simulink model "ex_ecg_sigprocessing"  (R2022b)
settings: Solver=VariableStepAuto  StartTime=0.0  StopTime=10  RelTol=1e-3  EnableMultiTasking=on
InitFcn:
  | % load recorded real (sampled from a healthy volunteer)
  | % and synthesized ECG data with Fs = 360 Hz
  | % Setting for generating the synthesized ECG data:
  | % Additive uniformly distributed measurement noise 0.005mV
  | % Standard deviation of heart rate [1 beat per minute]
  | 
  | load('ex_ecgdata360Hz.mat')
  | % ecgdata360Hz_hrmean45 : synthesized ECG signal with mean heart rate 45 bpm
  | % ecgdata360Hz_hrmean60 : synthesized ECG signal with mean heart rate 60 bpm
  | % ecgdata360Hz_hrmean160 : synthesized ECG signal with mean heart rate 160 bpm
  | % ecgdata360Hz_hrmean220 : synthesized ECG signal with mean heart rate 220 bpm
  | % ecgdata360Hz_hrmean82 : recorded real ECG sample from a healthy MathWorks volunteer
  | 
  | fs = 360; % sampling frequency of recorded ECG data Hz
  | 
  | 
  | % Define filter
  | fs_filter = 200; % sampling frequency of the filter
  | fc = [5 26]; % Bandpass Filter Spec [Hz]
  | 
  | fc_bandpass = fc/(1/2*fs_filter); % Normalized freq (Matlab convention)
  | 
  | %N = 256; % Order of filter
  | %b = fir1(N,fc_bandpass);
  | 
  | %
  | WinWidthMS = 80; % ms or 80 ms
  | WinSize = WinWidthMS*fs_filter/1000; % moving average window size 80ms
libraries: dspsrcs4 x5, dspsigops x1, dspfdesign x1, slpidlib x1, sldrtlib x1
CloseFcn:
  | clear fc;
  | clear fc_bandpass;
  | clear fs;
  | clear fs_filter;
  | clear WinWidthMS;
  | clear WinSize;
  | clear ecgdata360Hz_hrmean45;
  | clear ecgdata360Hz_hrmean60;
  | clear ecgdata360Hz_hrmean82;
  | clear ecgdata360Hz_hrmean160;
  | clear ecgdata360Hz_hrmean220;
settings Model: ExtModeTrigDuration=10000  Creator=The MathWorks, Inc.  LastModifiedBy={ AZAN Laptops }
settings SolverCC: AlgebraicLoopSolver=TrustRegion  MaxZcPerStep=1
settings DataIOCC: LimitDataPoints=on  SaveFormat=Array  ReturnWorkspaceOutputs=off
settings OptimizationCC: LifeSpan=1  MaxStackSize=64  SimCompilerOptimization=on  EfficientTunableParamExpr=on
settings DebuggingCC: SolverPrmCheckMsg=warning  ParameterPrecisionLossMsg=none  UnconnectedInputMsg=warning  UnconnectedOutputMsg=warning  UnconnectedLineMsg=warning  AllowSymbolicDim=off  SymbolicDimsDataTypeCodeGenerationDiagnostic=none  SFUnexpectedBacktrackingDiag=warning  SFNoUnconditionalDefaultTransitionDiag=warning  SFExecutionAtInitializationDiag=none  SFMachineParentedDataDiag=warning  ArithmeticOperatorsInVariantConditions=warning
settings HardwareCC: ProdBitPerPointer=32  ProdLargestAtomicInteger=Long  ProdLargestAtomicFloat=Double  ProdIntDivRoundTo=Undefined  ProdWordSize=32  ProdHWDeviceType=ARM Compatible->ARM Cortex
settings ModelReferenceCC: EnableRefExpFcnMdlSchedulingChecks=on  PropagateSignalLabelsOutOfModel=off
settings SFSimCC: SimUseLocalCustomCode=off  MATLABDynamicMemAlloc=off  CustomCodeUndefinedFunction=UseInterfaceOnly
settings RTWCC: Description=Embedded Coder  SystemTargetFile=ert.tlc  TemplateMakefile=ert_default_tmf  RTWUseLocalCustomCode=off  DLArmComputeVersion=19.05
settings CodeAppCC: IgnoreCustomStorageClasses=off  StateflowObjectComments=on
settings ERTTargetCC: MultiwordLength=2048  ERTCustomFileTemplate=example_file_process.tlc  ConvertIfToSwitch=off  SuppressUnreachableDefaultCases=off
settings ConfigComp: CovMetricSettings=dw  CovSaveCumulativeToWorkspaceVar=on  CovSaveSingleToWorkspaceVar=on  CovExternalEMLEnable=off  CovSFcnEnable=off

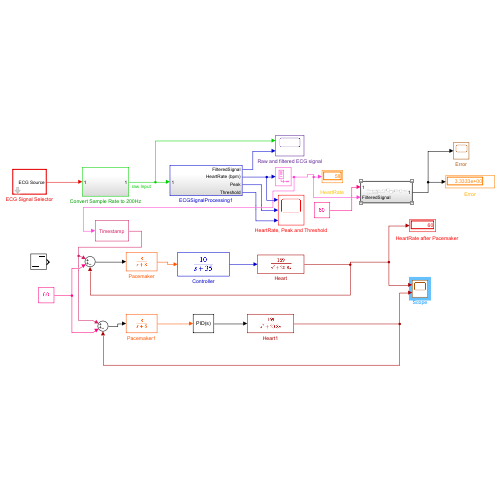
[thumbnail: Simulink's stored preview of the top-level diagram]
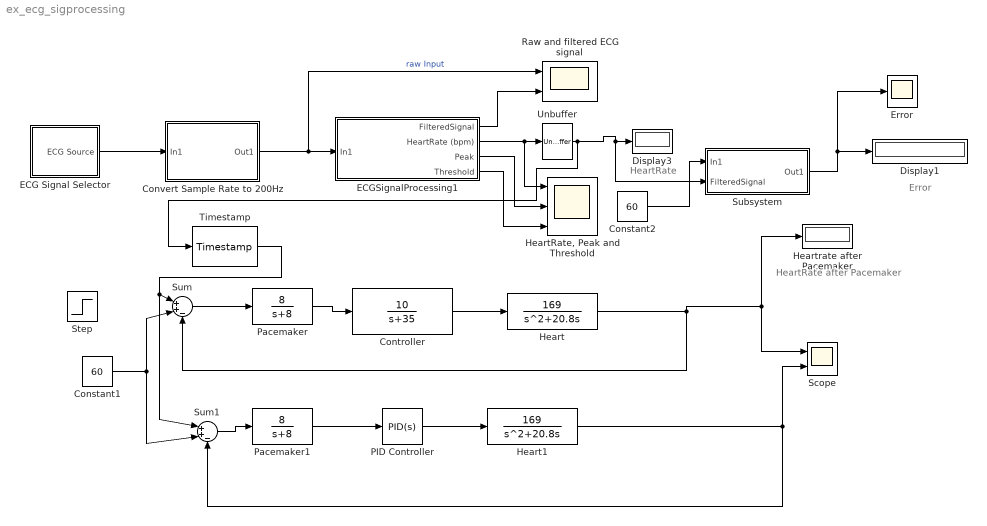
== system ex_ecg_sigprocessing ==
  note: HeartRate
  note: HeartRate after Pacemaker
  note: Error
  Constant1 : Constant  Value=60
  Constant2 : Constant  Value=60
  Controller : TransferFcn  Numerator=[10]  Denominator=[1 35]
  Convert Sample Rate to 200Hz : Subsystem
  Display1 : Display
      settings: Format=short_e
  Display3 : Display
  ECG Signal Selector : Subsystem  TreatAsAtomicUnit=on  mask{K=60 bpm (synthesized)}
      mask prompts: K "Select ECG Signal Mean Heart Rate (Beats Per Minute)"
      mask Help: web(fullfile(docroot,'dsp','examples','real-time-ecg-qrs-detection.html#zmw57dd0e14307'));
      mask TypeOptions K: 45 bpm (synthesized) | 60 bpm (synthesized) | 82 bpm (recorded) | 160 bpm (synthesized) | 220 bpm (synthesized)
  ECGSignalProcessing1 : Subsystem
  Error : Scope
  Heart : TransferFcn  Numerator=[169]  Denominator=[1 20.8 0]
  Heart1 : TransferFcn  Numerator=[169]  Denominator=[1 20.8 0]
  "HeartRate, Peak and Threshold" : Scope  NumInputPorts=3
  "Heartrate after Pacemaker " : Display
  PID Controller : slpidlib/PID Controller  Controller=PID  Form=Parallel  TimeDomain=Continuous-time  UseExternalTs=off  SampleTime=-1  IntegratorMethod=Forward Euler  FilterMethod=Forward Euler  ControllerParametersSource=internal  P=1  I=1  UseKiTs=off  D=0.1  N=100  UseFilter=on  TunerSelectOption=Transfer Function Based (PID Tuner App)  InitialConditionSource=internal  InitialConditionForIntegrator=0  InitialConditionForFilter=0  DifferentiatorICPrevScaledInput=0  ExternalReset=none  TrackingMode=off  Kt=1  LimitOutput=off  SatLimitsSource=internal  UpperSaturationLimit=inf  LowerSaturationLimit=-inf  LinearizeAsGain=on  AntiWindupMode=none  Kb=1  LimitIntegrator=off  UpperIntegratorSaturationLimit=inf  LowerIntegratorSaturationLimit=-inf  POutMin=[]  POutMax=[]  IOutMin=[]  IOutMax=[]  DOutMin=[]  DOutMax=[]  NOutMin=[]  NOutMax=[]  SumOutMin=[]  SumOutMax=[]  SaturationOutMin=[]  SaturationOutMax=[]  PParamMin=[]  PParamMax=[]  IParamMin=[]  IParamMax=[]  DParamMin=[]  DParamMax=[]  NParamMin=[]  NParamMax=[]  KbParamMin=[]  KbParamMax=[]  KtParamMin=[]  KtParamMax=[]  KbOutMin=[]  KbOutMax=[]  KtOutMin=[]  KtOutMax=[]  IntegratorOutMin=[]  IntegratorOutMax=[]  FilterOutMin=[]  FilterOutMax=[]  SumI1OutMin=[]  SumI1OutMax=[]  SumI2OutMin=[]  SumI2OutMax=[]  SumI3OutMin=[]  SumI3OutMax=[]  SumI4OutMin=[]  SumI4OutMax=[]  SumDOutMin=[]  SumDOutMax=[]  DifferentiatorOutMin=[]  DifferentiatorOutMax=[]  FilterDiffOutCoefMin=[]  FilterDiffOutCoefMax=[]  ReciprocalOutMin=[]  ReciprocalOutMax=[]  SumDenOutMin=[]  SumDenOutMax=[]  SumNumOutMin=[]  SumNumOutMax=[]  DivideOutMin=[]  DivideOutMax=[]  UdiffTsProdOutMin=[]  UdiffTsProdOutMax=[]  NTsProdOutMin=[]  NTsProdOutMax=[]  UintegralTsProdOutMin=[]  UintegralTsProdOutMax=[]  UngainTsProdOutMin=[]  UngainTsProdOutMax=[]  ClampingZeroOutDataTypeStr=Inherit: Inherit via back propagation  ClampingZeroOutMin=[]  ClampingZeroOutMax=[]  FilterDenConstantOutDataTypeStr=Inherit: Inherit via back propagation  FilterDenConstantOutMin=[]  FilterDenConstantOutMax=[]  PCopyOutDataTypeStr=Inherit: Inherit via back propagation  PCopyOutMin=[]  PCopyOutMax=[]  NCopyOutDataTypeStr=Inherit: Inherit via back propagation  NCopyOutMin=[]  NCopyOutMax=[]  IntegratorContinuousStateAttributes=''  IntegratorStateMustResolveToSignalObject=off  IntegratorRTWStateStorageClass=Auto  FilterContinuousStateAttributes=''  FilterStateMustResolveToSignalObject=off  FilterRTWStateStorageClass=Auto  ParallelPVariant=InternalParameters  IdealPVariant=Disabled  IVariant=InternalParameters  DVariant=InternalParameters  IntegratorVariant=Continuous  SatVariant=Disabled  AWVariant=Passthrough  PCopyVariant=Disabled  TRVariant=Disabled  FdbkBlocksVariant=Forward  IdealPFdbkVariant=Disabled  SatFdbkVariant=Disabled  DerivativeFilterVariant=ContFilter  NVariant=InternalParameters  NCopyVariant=Disabled  FilterICVariant=InternalICsFilter  IntegratorICVariant=InternalICs  ExternalResetVariant=Disabled  TRSumVariant=Passthrough  SumFdbkVariant=Disabled  SumVariant=Sum_PID  TsampFilterVariant=InternalTs  TsampNgainVariant=Passthrough  TsampIntegralVariant=Passthrough  ExternalSaturationOutDataTypeStr=Inherit: Same as second input
  Pacemaker : TransferFcn  Numerator=[8]  Denominator=[1 8]
  Pacemaker1 : TransferFcn  Numerator=[8]  Denominator=[1 8]
  Raw and filtered ECG signal : Scope  NumInputPorts=2
  Scope : Scope  NumInputPorts=2
  Step : Step  SampleTime=0
  Subsystem : Subsystem
  Sum : Sum  Inputs=|++-
  Sum1 : Sum  Inputs=|++-
  Timestamp : sldrtlib/Target Profiling/Timestamp
  Unbuffer : Unbuffer
  wires:
  ECGSignalProcessing1/2(HeartRate (bpm)) -> "HeartRate, Peak and Threshold"/1, Unbuffer/1
  ECGSignalProcessing1/1(FilteredSignal) -> Raw and filtered ECG signal/2
  ECGSignalProcessing1/3(Peak) -> "HeartRate, Peak and Threshold"/2
  ECGSignalProcessing1/4(Threshold) -> "HeartRate, Peak and Threshold"/3
  ECG Signal Selector/1(ECG Source) -> Convert Sample Rate to 200Hz/1(In1)
  Convert Sample Rate to 200Hz/1(Out1) -> ECGSignalProcessing1/1(In1), Raw and filtered ECG signal/1  "raw Input"
  Constant1/1 -> Sum1/2, Sum/2
  Heart/1 -> "Heartrate after Pacemaker "/1, Scope/1, Sum/3
  Sum/1 -> Pacemaker/1
  Unbuffer/1 -> Timestamp/1, Subsystem/2(FilteredSignal), Display3/1
  Subsystem/1(Out1) -> Display1/1, Error/1
  Constant2/1 -> Subsystem/1(In1)
  Controller/1 -> Heart/1
  Pacemaker/1 -> Controller/1
  PID Controller/1 -> Heart1/1
  Pacemaker1/1 -> PID Controller/1
  Sum1/1 -> Pacemaker1/1
  Heart1/1 -> Sum1/3, Scope/2
  Timestamp/1 -> Sum1/1, Sum/1

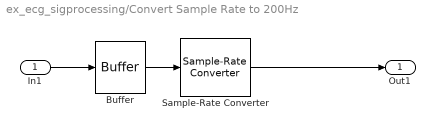
== system ex_ecg_sigprocessing/Convert Sample Rate to 200Hz ==
  In1 : Inport
  Buffer : Buffer  N=90
  Sample-Rate Converter : dspsigops/Sample-Rate Converter  InputSampleRate=fs  OutputSampleRate=200  OutputRateTolerance=0.01  Bandwidth=198  StopbandAttenuation=60  SimulateUsing=Code generation
  Out1 : Outport  VectorParamsAs1DForOutWhenUnconnected=off
  wires:
  In1/1 -> Buffer/1
  Sample-Rate Converter/1 -> Out1/1
  Buffer/1 -> Sample-Rate Converter/1

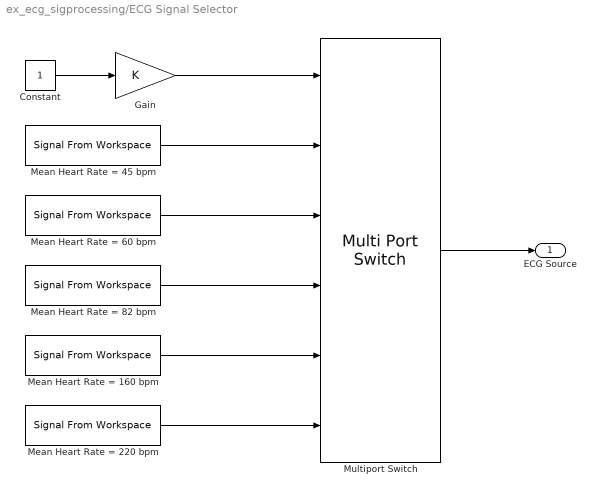
== system ex_ecg_sigprocessing/ECG Signal Selector ==
  " Mean Heart Rate = 160 bpm" : dspsrcs4/Signal From Workspace  X=ecgdata360Hz_hrmean160  Ts=1/fs  nsamps=1  OutputAfterFinalValue=Cyclic repetition  ignoreOrWarnInputAndFrameLengths=off  OutputFrames=on
  " Mean Heart Rate = 220 bpm" : dspsrcs4/Signal From Workspace  X=ecgdata360Hz_hrmean220  Ts=1/fs  nsamps=1  OutputAfterFinalValue=Cyclic repetition  ignoreOrWarnInputAndFrameLengths=off  OutputFrames=on
  " Mean Heart Rate = 45 bpm" : dspsrcs4/Signal From Workspace  X=ecgdata360Hz_hrmean45  Ts=1/fs  nsamps=1  OutputAfterFinalValue=Cyclic repetition  ignoreOrWarnInputAndFrameLengths=off  OutputFrames=on
  " Mean Heart Rate = 60 bpm " : dspsrcs4/Signal From Workspace  X=ecgdata360Hz_hrmean60  Ts=1/fs  nsamps=1  OutputAfterFinalValue=Cyclic repetition  ignoreOrWarnInputAndFrameLengths=off  OutputFrames=on
  " Mean Heart Rate = 82 bpm" : dspsrcs4/Signal From Workspace  X=ecgdata360Hz_hrmean82  Ts=1/fs  nsamps=1  OutputAfterFinalValue=Cyclic repetition  ignoreOrWarnInputAndFrameLengths=off  OutputFrames=on
  Constant : Constant
  Gain : Gain  Gain=K
  Multiport Switch : MultiPortSwitch  Inputs=5  OutDataTypeStr=single  SaturateOnIntegerOverflow=off  InputSameDT=off
  ECG Source : Outport  VectorParamsAs1DForOutWhenUnconnected=off
  wires:
  Gain/1 -> Multiport Switch/1
  Constant/1 -> Gain/1
  Multiport Switch/1 -> ECG Source/1
  " Mean Heart Rate = 45 bpm"/1 -> Multiport Switch/2
  " Mean Heart Rate = 60 bpm "/1 -> Multiport Switch/3
  " Mean Heart Rate = 82 bpm"/1 -> Multiport Switch/4
  " Mean Heart Rate = 160 bpm"/1 -> Multiport Switch/5
  " Mean Heart Rate = 220 bpm"/1 -> Multiport Switch/6

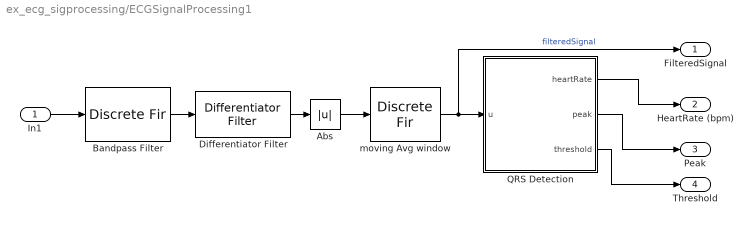
== system ex_ecg_sigprocessing/ECGSignalProcessing1 ==
  In1 : Inport
  Abs : Abs  SaturateOnIntegerOverflow=off
  Bandpass Filter : DiscreteFir  DialogController=Simulink.DDGSource  Coefficients=fir1(256,fc_bandpass)  InputProcessing=Columns as channels (frame based)
  Differentiator Filter : dspfdesign/Differentiator Filter  DesignForMinimumOrder=off  FilterOrder=51  PassbandRipple=0.1  ScaleCoefficients=off  SimulateUsing=Interpreted execution  roundingMode=Floor  coeffsDataTypeStr=fixdt(1,16)
  QRS Detection : MATLAB Function  TreatAsAtomicUnit=on
  moving Avg window : DiscreteFir  DialogController=Simulink.DDGSource  Coefficients=ones(1, WinSize, 'single')/WinSize  InputProcessing=Columns as channels (frame based)
  FilteredSignal : Outport  VectorParamsAs1DForOutWhenUnconnected=off
  HeartRate (bpm) : Outport  Port=2  VectorParamsAs1DForOutWhenUnconnected=off
  Peak : Outport  Port=3  VectorParamsAs1DForOutWhenUnconnected=off
  Threshold : Outport  Port=4  VectorParamsAs1DForOutWhenUnconnected=off
  wires:
  moving Avg window/1 -> QRS Detection/1(u), FilteredSignal/1  "filteredSignal"
  In1/1 -> Bandpass Filter/1
  QRS Detection/2(peak) -> Peak/1
  QRS Detection/3(threshold) -> Threshold/1
  Abs/1 -> moving Avg window/1
  Bandpass Filter/1 -> Differentiator Filter/1
  QRS Detection/1(heartRate) -> HeartRate (bpm)/1
  Differentiator Filter/1 -> Abs/1

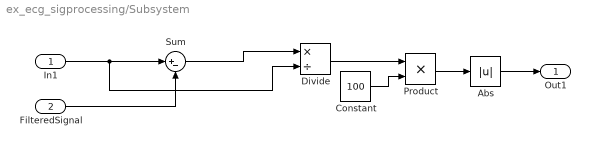
== system ex_ecg_sigprocessing/Subsystem ==
  In1 : Inport
  FilteredSignal : Inport  Port=2
  Abs : Abs  SaturateOnIntegerOverflow=off
  Constant : Constant  Value=100
  Divide : Product  Inputs=*/
  Product : Product
  Sum : Sum  Inputs=|+-
  Out1 : Outport
  wires:
  In1/1 -> Divide/2, Sum/1
  FilteredSignal/1 -> Sum/2
  Sum/1 -> Divide/1
  Divide/1 -> Product/1
  Constant/1 -> Product/2
  Product/1 -> Abs/1
  Abs/1 -> Out1/1

== matlab function ex_ecg_sigprocessing/ECGSignalProcessing1/QRS Detection ==
  data: heartRate output; peak output; u input; threshold output
function [heartRate,peak,threshold]  = QRSDetection(u)

    persistent FS QRSDelay
    if isempty(FS)
        FS = 200; % Hz, samples per second
        QRSDelay = zeros(size(u), 'like', u);
    end
    
    heartRate = uint16(zeros(size(u)));
    peak = zeros(size(u), 'like', u);    
    threshold = zeros(size(u), 'like', u);
    % Prevents detections of peaks smaller than 150 uV.
    MIN_PEAK_AMP = cast(7/2^12, 'like', u(1));

    for idx = 1:length(u) 
        % For a frame of input signal, process one sample at a time
        peak(idx) = findpeak(u(idx));

        if(peak(idx) < MIN_PEAK_AMP)
            peak(idx) = 0 ;
        end

        % returns adjusted peak
        [QRSDelay(idx), threshold(idx), peak(idx)] = qrs_det(peak(idx));
        if QRSDelay(idx) ~= 0
            % beat per min = samplesPerSec * 60sec/min / samples per beat_oneQRSDalay
            heartRate(idx) = int16(60 * FS / QRSDelay(idx));
        end

    end
end % function QRSDetection


function pk = findpeak(datum)
    % peak() takes a datum as input and returns a peak height
    % when the signal returns to half its peak height, or it has been
    % 95 ms since the peak height was detected.
    
    persistent maxPeak lastDatum timeSinceMax
    pk = cast(0,'like',datum);
    if isempty(maxPeak)
        maxPeak = cast(0,'like',datum);
        lastDatum = cast(0,'like',datum);
        timeSinceMax = uint16(0);
        return
    end
    
    if timeSinceMax > 0
        timeSinceMax(:) = timeSinceMax + 1;
    end
    
    if((datum > lastDatum) && (datum > maxPeak)) % rising slope
        maxPeak(:) = datum ;
        if(maxPeak > 2) % reset timeSinceMax 
            timeSinceMax(:) = 1 ;
        end
    elseif(datum < bitsra(maxPeak,1)) % middle of falling slope
        % Less than half the peak height
        pk(:) = maxPeak ;
        maxPeak(:) = 0 ;
        timeSinceMax(:) = 0 ;
    elseif(timeSinceMax > MS95)
        pk(:) = maxPeak ;
        maxPeak(:) = 0 ;
        timeSinceMax(:) = 0 ;
    end
    lastDatum = datum ;
end

function [QRSDelay,thisThreshold, pk] = qrs_det(pk)
    
    persistent count 
    persistent qpkcnt
    persistent lastQRSDelay
    persistent threshold
    persistent preBlankCnt
    persistent tempPeak
    persistent initMax
    persistent sbpeak
    persistent sbcount
        
    if isempty(lastQRSDelay)
        count = int16(0);
        qpkcnt = int16(0);
        lastQRSDelay = int16(0);
        % EC13: QRS detector should not detect QRS complexes with 
        %  amplitudes of less than 0.15mV and 1mV QRS complexes with width
        %  less than 10ms (6000bpm)
        threshold = cast(8/2^12, 'like', pk);
        tempPeak = cast(0, 'like', pk);
        initMax = cast(0, 'like', pk);
        preBlankCnt = int16(0);
        sbpeak = cast(0, 'like', pk);
        sbcount = int16(MS1650);
    end
    
    % there can only be one QRS complex in any 196ms (306bpm) window
    if (pk==0) && (preBlankCnt==0)
        pk(:) = 0;
    elseif (pk==0) && (preBlankCnt~=0)
        % if we have held onto a peak for 196ms, pass it on for eval
        preBlankCnt = preBlankCnt - 1;
        if (preBlankCnt == 0)
            pk(:) = tempPeak;
        else
            pk(:) = 0;
        end        
    elseif (pk~=0) && (preBlankCnt==0)
        % if there has been no peak for 196ms, save this one and start
        % counting
        tempPeak = pk;
        preBlankCnt = MS196;
        pk(:) = 0;
    else % (pk~=0) &&  (preBlankCnt~=0)
        % if we were holding a peak, but this one is bigger,
        % save it and start counting to 196ms again
        if (pk > tempPeak)
            tempPeak = pk;
            preBlankCnt = MS196;
            pk(:) = 0;
        else
            preBlankCnt = preBlankCnt - 1;
            if (preBlankCnt == 0)
                pk(:) = tempPeak;
            else
                pk(:) = 0;
            end
        end
    end
    
    count(:) = count + 1;
    
    % Initialize the QRS peak buffer with the first eight 
    % local maximum peaks detected
    if qpkcnt < 8
        if pk > 0
           UPDATEQ = true;
           threshold = updateQN(pk, UPDATEQ);
           qpkcnt = qpkcnt + 1;
           if pk > initMax 
               initMax = pk;
           end
           if qpkcnt == 8
               count(:) = 0;
           end
           
        end
        
    else % qpkcnt >= 8
        
        if pk > threshold
            UPDATEQ = true;
            threshold = updateQN(pk, UPDATEQ);
            lastQRSDelay(:) = count;
            count(:) = 0;
            sbpeak(:) = 0;
        elseif pk ~= 0
            % if peak is below threshold
            UPDATEQ = false;
            threshold = updateQN(pk, UPDATEQ);
            
            % If no QRS has been detected within 1.5 R-to-R intervals, 
            % there was a peak that was larger than half the 
            % detection threshold, and the peak followed the preceding 
            % detection by at least 360ms, classify that peak as a QRS 
            % complex
            
            % persistent sbpeak = 0; sbcount = MS1650
            if (count >= MS360) && (pk > sbpeak)
                sbpeak = pk;
                sbloc = count;
                threshold(:) = bitsra(threshold,1);
                
                if (count > sbcount) && (sbpeak > threshold)
                    sbcount = updateRR(sbloc);
                    lastQRSDelay(:) = count;
                    % threshold = threshold >> 1;
                    count(:) = 0;
                    sbpeak(:) = 0;
                end
            end
            
        end
    end
    QRSDelay = lastQRSDelay;
    thisThreshold = threshold;
end


function det_thresh = updateQN(x, Qflag)
  persistent QSum
  persistent NSum
  persistent Qz Nz nQ nN

  if isempty(NSum)
      nQ = uint8(0);
      nN = uint8(0);
      Qz = zeros(8,1,'like',x);
      Nz = zeros(8,1,'like',x);
      QSum = cast(0, 'like', x);
      NSum = cast(0, 'like', x);
  end

  det_thresh = cast(0, 'like', x);
  if Qflag %&& x ~= cast(0,'like',x)
      Qz(nQ+1) = x;
      nQ = bitand(nQ+1,uint8(7));
      QSum(:) = sum(Qz);
  else
      Nz(nN+1) = x;
      nN = bitand(nN+1,uint8(7));
      NSum(:) = sum(Nz);
  end
  det_thresh(:) = QSum-NSum ;
  det_thresh(:) = NSum + bitsra(det_thresh,1) - bitsra(det_thresh,3);
  det_thresh(:) = bitsra(det_thresh, 3);
end

%**************************************************************************
%  UpdateRR takes a new RR value and updates the RR mean estimate
%*************************************************************************/
function sbcount = updateRR(x)
  persistent RRSum
  persistent zR 
  persistent nR

  if isempty(RRSum)
      nR = uint8(0);
      zR = cast(MS1000*ones(8,1, 'int16'),'like',x);
      RRSum = cast(bitsll(MS1000,3), 'like', x);
  end
  
  sbcount = cast(0, 'like', x);
  zR(nR+1) = x;
  nR = bitand(nR+1,uint8(7));
  RRSum(:) = sum(bitsra(zR,3));
  
  sbcount(:) = RRSum + bitsra(RRSum, 1); % = 1.5RRSum
  sbcount(:) = bitsra(sbcount, 3);
  sbcount(:) = sbcount + MS80; % WINDOW_WIDTH
end

function n = MS80
% The number of samples in 95 milli-seconds, where FS is the sample rate
    FS = 200;
    n = int16(80 * FS / 1000);
end

function n = MS95
% The number of samples in 95 milli-seconds, where FS is the sample rate
    FS = 200;
    n = int16(95 * FS / 1000);
end

function n = MS196
% The number of samples in 196 milli-seconds, where FS is the sample rate
    FS = 200;
    n = int16(196 * FS / 1000);
end

function n = MS360
% The number of samples in 360 milli-seconds, where FS is the sample rate
    FS = 200;
    n = int16(360 * FS / 1000);
end

function n = MS1000
% The number of samples in 1000 milli-seconds, where FS is the sample rate
    FS = 200;
    n = int16(1000 * FS / 1000);
end

function n = MS1650
% The number of samples in 1650 milli-seconds, where FS is the sample rate
    FS = 200;
    n = int16(1650 * FS / 1000);
end
